simulink model "s3"  (Simulink 2.00)
settings: Solver=ode45  StartTime=0.0  StopTime=0.95  MaxStep=1e-3  RelTol=1e-6  AbsTol=1e-6
values from neighbouring files (symbols this model uses):
  alpha = input('Enter attenuation factor, alpha > ')    [M2.M]    (also in M3.M = input('Enter attenuation factor alpha, try 1,  > '))
  m = input('Enter value of m  > ')    [M2.M]    (also in M3.M = input('Enter the value of m for abc currents  > '))
  nframe = input('Enter the value of nframe of the qd0 frame  > ')    [M3.M]
  theta0 = input('Enter value of theta0 > ')    [M3.M]
settings Model: SaveTime=off  SaveOutput=off  ConsistencyChecking=off

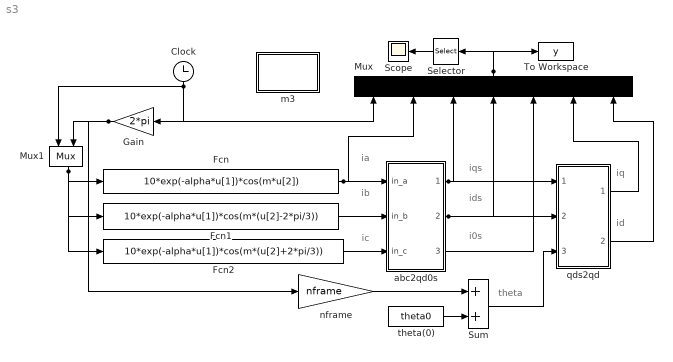
== system s3 ==
  note: iq
  note: id
  note: theta
  note: ic
  note: ia
  note: ib
  note: iqs
  note: ids
  note: i0s
  Clock : Clock
      settings: Orientation=down  DeleteFcn=simclock BlockIsBeingDestroyed  PostSaveFcn=simclock Save
  Fcn : Fcn  Expr=10*exp(-alpha*u[1])*cos(m*u[2])
  Fcn1 : Fcn  Expr=10*exp(-alpha*u[1])*cos(m*(u[2]-2*pi/3))
  Fcn2 : Fcn  Expr=10*exp(-alpha*u[1])*cos(m*(u[2]+2*pi/3))
  Gain : Gain  Orientation=left  Gain=2*pi
  m3 : Subsystem
      settings: OpenFcn=m3
      mask Type: Masked block of m3.m
      mask Help: Uses m3.m to initialize and plot
      mask Display: disp('Initialize\nand plot')
  Mux : Mux  Orientation=up  Inputs=7
  Mux1 : Mux  Orientation=down  Inputs=2
  Scope : Scope
      settings: TickLabels=on  TimeRange=1  YMin=-25  YMax=25  SaveToWorkspace=off  SaveName=ScopeData  Decimation=2
  Selector : Selector  Orientation=left  Elements=[1 2 3 4 5 6]  InputPortWidth=7
  Sum : Sum  Inputs=++
  To Workspace : ToWorkspace  VariableName=y  SampleTime=0
      settings: Buffer=10000
  abc2qd0s : Subsystem
  nframe : Gain  Gain=nframe
  qds2qd : Subsystem
  theta(0) : Constant  Value=theta0
  wires:
  Mux/1 -> Selector/1, To Workspace/1
  Selector/1 -> Scope/1
  Gain/1 -> nframe/1, Mux1/2
  Mux1/1 -> Fcn2/1, Fcn1/1, Fcn/1
  Clock/1 -> Mux1/1, Gain/1, Mux/1
  abc2qd0s/1(out_qs) -> qds2qd/1(in_qs), Mux/3
  theta(0)/1 -> Sum/2
  Sum/1 -> qds2qd/3("theta ")
  nframe/1 -> Sum/1
  qds2qd/2(out_d) -> Mux/7
  qds2qd/1(out_q) -> Mux/6
  abc2qd0s/3(out_0s) -> Mux/5
  abc2qd0s/2(out_ds) -> qds2qd/2(in_ds), Mux/4
  Fcn/1 -> Mux/2, abc2qd0s/1(in_a)
  Fcn2/1 -> abc2qd0s/3(in_c)
  Fcn1/1 -> abc2qd0s/2(in_b)

== system s3/m3 ==
  note: Masked block of m3.m

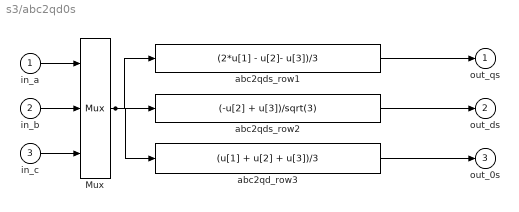
== system s3/abc2qd0s ==
  in_a : Inport  Port=1  PortWidth=-1  SampleTime=-1
  in_b : Inport  Port=2  PortWidth=-1  SampleTime=-1
  in_c : Inport  Port=3  PortWidth=-1  SampleTime=-1
  Mux : Mux  Inputs=3
  abc2qd_row3 : Fcn  Expr=(u[1] + u[2] + u[3])/3
  abc2qds_row1 : Fcn  Expr=(2*u[1] - u[2]- u[3])/3
  abc2qds_row2 : Fcn  Expr=(-u[2] + u[3])/sqrt(3)
  out_qs : Outport  Port=1  InitialOutput=0
  out_ds : Outport  Port=2  InitialOutput=0
  out_0s : Outport  Port=3  InitialOutput=0
  wires:
  Mux/1 -> abc2qd_row3/1, abc2qds_row2/1, abc2qds_row1/1
  abc2qd_row3/1 -> out_0s/1
  abc2qds_row2/1 -> out_ds/1
  abc2qds_row1/1 -> out_qs/1
  in_c/1 -> Mux/3
  in_b/1 -> Mux/2
  in_a/1 -> Mux/1

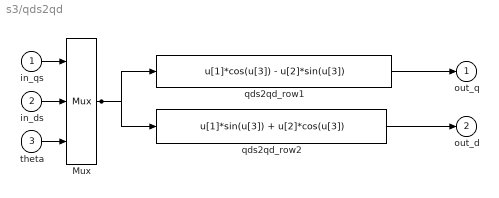
== system s3/qds2qd ==
  in_qs : Inport  Port=1  PortWidth=-1  SampleTime=-1
  in_ds : Inport  Port=2  PortWidth=-1  SampleTime=-1
  "theta " : Inport  Port=3  PortWidth=-1  SampleTime=-1
  Mux : Mux  Inputs=3
  qds2qd_row1 : Fcn  Expr=u[1]*cos(u[3]) - u[2]*sin(u[3])
  qds2qd_row2 : Fcn  Expr=u[1]*sin(u[3]) + u[2]*cos(u[3])
  out_q : Outport  Port=1  InitialOutput=0
  out_d : Outport  Port=2  InitialOutput=0
  wires:
  Mux/1 -> qds2qd_row1/1, qds2qd_row2/1
  "theta "/1 -> Mux/3
  in_ds/1 -> Mux/2
  in_qs/1 -> Mux/1
  qds2qd_row1/1 -> out_q/1
  qds2qd_row2/1 -> out_d/1
